simulink model "modelo_p1_2014_2"  (R2025a)
settings: Solver=VariableStepAuto  StartTime=0.0  StopTime=10.0  RelTol=1e-3
libraries: simulink x1
settings Model: Creator=joaof  LastModifiedBy=joaof

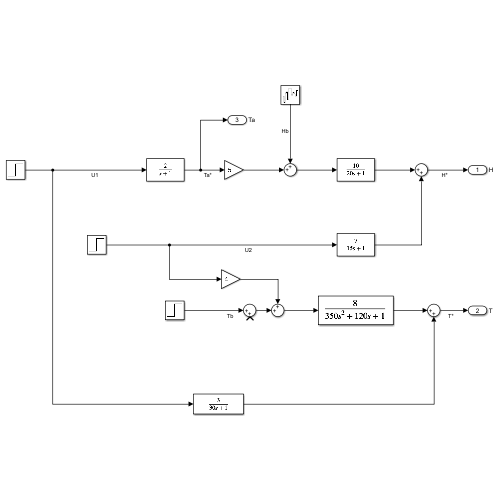
[thumbnail: Simulink's stored preview of the top-level diagram]
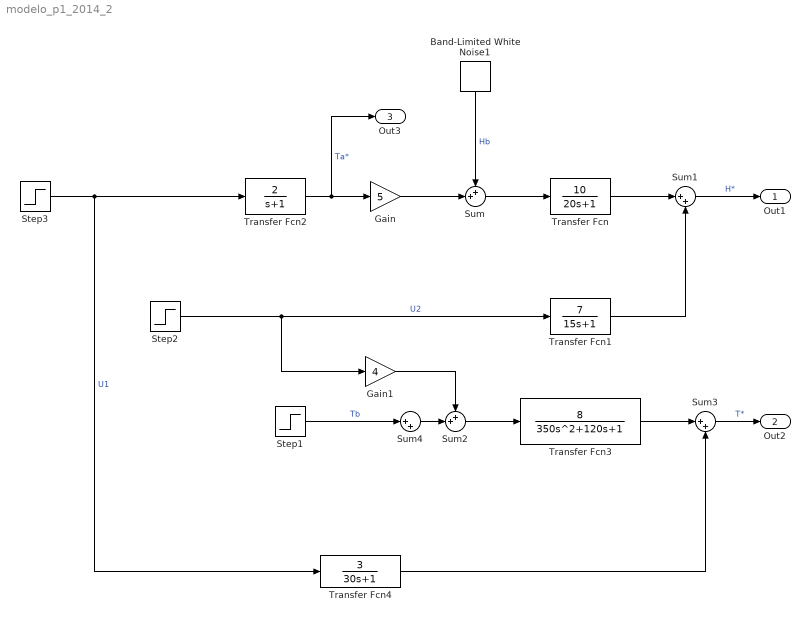
== system modelo_p1_2014_2 ==
  Band-Limited White Noise1 : simulink/Sources/Band-Limited White Noise  Cov=[0.1]  Ts=0.1  seed=[23341]
  Gain : Gain  Gain=5
  Gain1 : Gain  Gain=4
  Step1 : Step  SampleTime=0
  Step2 : Step  SampleTime=0
  Step3 : Step  SampleTime=0
  Sum : Sum  Inputs=++|
  Sum1 : Sum  Inputs=|++
  Sum2 : Sum  Inputs=++|
  Sum3 : Sum  Inputs=|++
  Sum4 : Sum  Inputs=|++
  Transfer Fcn : TransferFcn  Numerator=[10]  Denominator=[20 1]
  Transfer Fcn1 : TransferFcn  Numerator=[7]  Denominator=[15 1]
  Transfer Fcn2 : TransferFcn  Numerator=[2]  Denominator=[1 1]
  Transfer Fcn3 : TransferFcn  Numerator=[8]  Denominator=[350 120 1]
  Transfer Fcn4 : TransferFcn  Numerator=[3]  Denominator=[30 1]
  Out1 : Outport  SignalName=H
  Out2 : Outport  Port=2  SignalName=T
  Out3 : Outport  Port=3  SignalName=Ta
  wires:
  Gain/1 -> Sum/2
  Sum/1 -> Transfer Fcn/1
  Band-Limited White Noise1/1 -> Sum/1  "Hb"
  Step2/1 -> Gain1/1, Transfer Fcn1/1  "U2"
  Transfer Fcn2/1 -> Out3/1, Gain/1  "Ta*"
  Step3/1 -> Transfer Fcn2/1, Transfer Fcn4/1  "U1"
  Transfer Fcn1/1 -> Sum1/2
  Transfer Fcn/1 -> Sum1/1
  Sum1/1 -> Out1/1  "H*"
  Step1/1 -> Sum4/1  "Tb"
  Gain1/1 -> Sum2/1
  Sum2/1 -> Transfer Fcn3/1
  Transfer Fcn3/1 -> Sum3/1
  Sum3/1 -> Out2/1  "T*"
  Transfer Fcn4/1 -> Sum3/2
  Sum4/1 -> Sum2/2
